simulink model "mpc_nonlinear"  (Simulink 6.0)
settings: Solver=ode45  SolverMode=SingleTasking  StartTime=0.0  StopTime=Tfinal  RelTol=1e-3
libraries: mpclib x1
settings Model: Creator=jowen  LastModifiedBy=Xbemporad  ExtModeTrigMode=oneshot  ExtModeArmWhenConnect=off
settings DataIOCC: LimitDataPoints=off  SignalLoggingName=sigsOut
settings OptimizationCC: BooleanDataType=off
settings DebuggingCC: CheckExecutionContextPreStartOutputMsg=on  CheckExecutionContextRuntimeOutputMsg=on  SolverPrmCheckMsg=none  IntegerOverflowMsg=none
settings HardwareCC: TargetUnknown=on
settings GRTTargetCC: ModelReferenceCompliant=off  MatFileLogging=off

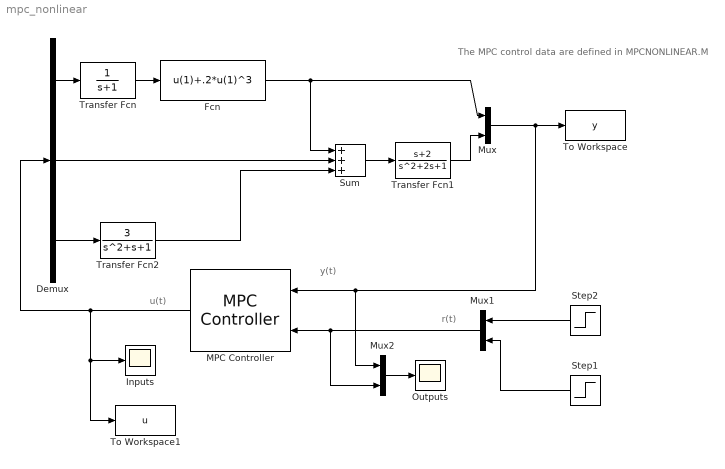
== system mpc_nonlinear ==
  note: u(t)
  note: y(t)
  note: r(t)
  note: The MPC control data are
      | defined in MPCNONLINEAR.M
  Demux : Demux  Outputs=3
  Fcn : Fcn  Expr=u(1)+.2*u(1)^3
  Inputs : Scope
      settings: TimeRange=8  YMin=-1  YMax=2  DataFormat=Structure
  MPC Controller : mpclib/MPC Controller  Orientation=left  mpcobj=MPCobj  n_mv=0  x0=[]  ref_from_ws=off  ref_signal_name=[]  ref_preview=on  md_from_ws=off  md_signal_name=[]  md_preview=on  from_project=off  md_inport=off  project_file=MPCtask.mat
  Mux : Mux  Inputs=2
  Mux1 : Mux  Orientation=left  Inputs=2
  Mux2 : Mux  Inputs=2
  Outputs : Scope
      settings: TimeRange=8  YMin=-0.5  YMax=1.5  DataFormat=Structure
  Step1 : Step  Orientation=left  Time=0  SampleTime=0
  Step2 : Step  Orientation=left  Time=2  SampleTime=0
  Sum : Sum  Inputs=+++  SaturateOnIntegerOverflow=on  InputSameDT=on
  To Workspace : ToWorkspace  VariableName=y  SampleTime=-1  SaveFormat=Array
      settings: MaxDataPoints=Inf
  To Workspace1 : ToWorkspace  VariableName=u  SampleTime=-1  SaveFormat=Array
      settings: MaxDataPoints=Inf
  Transfer Fcn : TransferFcn  Denominator=[1 1]
  Transfer Fcn1 : TransferFcn  Numerator=[1 2]
  Transfer Fcn2 : TransferFcn  Numerator=[3]  Denominator=[1 1 1]
  wires:
  MPC Controller/1 -> Demux/1, To Workspace1/1, Inputs/1
  Mux/1 -> To Workspace/1, Mux2/1, MPC Controller/1
  Demux/3 -> Transfer Fcn2/1
  Transfer Fcn2/1 -> Sum/3
  Transfer Fcn/1 -> Fcn/1
  Fcn/1 -> Sum/1, Mux/1
  Demux/2 -> Sum/2
  Sum/1 -> Transfer Fcn1/1
  Demux/1 -> Transfer Fcn/1
  Transfer Fcn1/1 -> Mux/2
  Step1/1 -> Mux1/2
  Mux1/1 -> Mux2/2, MPC Controller/2
  Step2/1 -> Mux1/1
  Mux2/1 -> Outputs/1
